simulink model "rtwdemo_advisor3"  (Simulink 7.6)
settings: Solver=FixedStepDiscrete  SolverMode=SingleTasking  StartTime=0.0  StopTime=4  FixedStep=1  RelTol=1e-3  AbsTol=1e-6
libraries: rtwdemowidgets x1
Description:
  | Using Model Advisor for optimizing the model for real-time deployment
settings Model: Creator=The MathWorks Inc.  CovMetricSettings=d  ExtModeTrigMode=oneshot  ExtModeArmWhenConnect=off  ExtModeAutoUpdateStatusClock=off
settings MATStruct: SampleTime=1  Offset=0  Priority=[20.0]
settings DataIOCC: LimitDataPoints=off  SaveOutput=off  SaveTime=off  SignalLoggingName=sigsOut
settings OptimizationCC: InlineParams=on  InlineInvariantSignals=on  PassReuseOutputArgsAs=Individual arguments  ZeroExternalMemoryAtStartup=off  ZeroInternalMemoryAtStartup=off  NoFixptDivByZeroProtection=on  EfficientFloat2IntCast=on  EfficientMapNaN2IntZero=off  OptimizeModelRefInitCode=on  LifeSpan=1
settings DebuggingCC: CheckExecutionContextPreStartOutputMsg=on  CheckExecutionContextRuntimeOutputMsg=on  SolverPrmCheckMsg=none  IntegerOverflowMsg=none  ParameterDowncastMsg=warning  ParameterOverflowMsg=warning  ParameterPrecisionLossMsg=none  StrictBusMsg=ErrorOnBusTreatedAsVector
settings HardwareCC: ProdIntDivRoundTo=Zero  ProdEndianess=LittleEndian  ProdHWDeviceType=Generic->32-bit Embedded Processor  TargetHWDeviceType=Generic->32-bit Embedded Processor
settings RTWCC: SystemTargetFile=ert.tlc  GenCodeOnly=on  TemplateMakefile=ert_default_tmf  GenerateReport=on  RTWVerbose=off  ProcessScript=ert_make_rtw_hook  IncludeHyperlinkInReport=on  LaunchReport=on
settings CodeAppCC: IgnoreCustomStorageClasses=off  IgnoreTestpoints=on  IncHierarchyInIds=on  IncDataTypeInIds=on
settings ERTTargetCC: TargetFcnLib=ansi_tfl_tmw.mat  MultiwordLength=2048  GenerateSampleERTMain=on  SupportNonFinite=off  ERTCustomFileTemplate=example_file_process.tlc  ConvertIfToSwitch=off

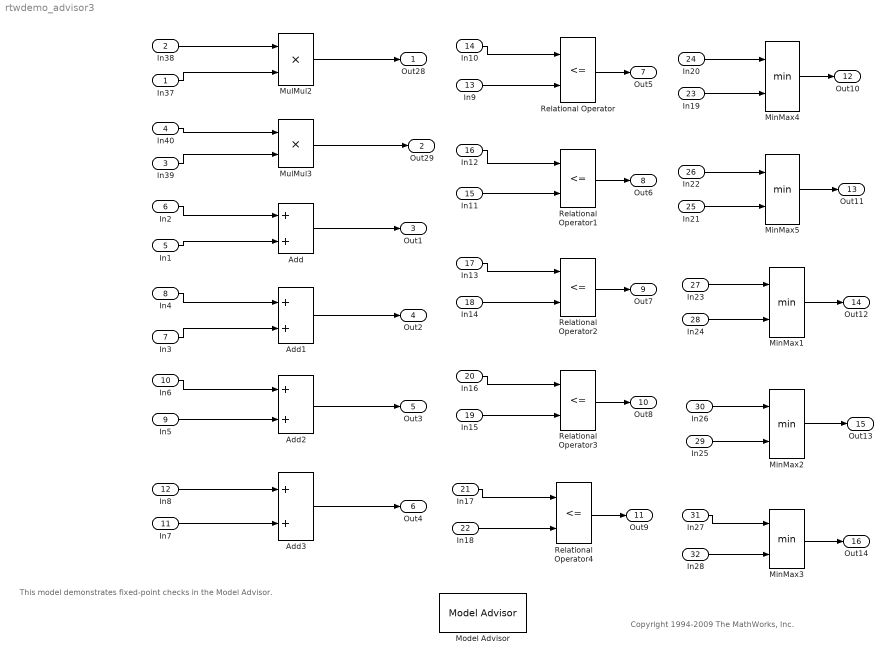
== system rtwdemo_advisor3 ==
  note: This model demonstrates fixed-point
      | checks in the Model Advisor.
  note: Copyright 1994-2009 The MathWorks, Inc.
  In37 : Inport  OutDataTypeStr=fixdt(1, 16, 1.375*2^-10, 0)  PortDimensions=1  SampleTime=1  Interpolate=off
  In38 : Inport  Port=2  OutDataTypeStr=fixdt(1, 16, 1.25 * 2^-10, 0)  PortDimensions=1  SampleTime=1  Interpolate=off
  In39 : Inport  Port=3  OutDataTypeStr=fixdt(1,16,10)  PortDimensions=1  SampleTime=1  Interpolate=off
  In40 : Inport  Port=4  OutDataTypeStr=fixdt(1, 16, 2^-10,1)  PortDimensions=1  SampleTime=1  Interpolate=off
  In1 : Inport  Port=5  OutDataTypeStr=fixdt(1,8,5)  PortDimensions=1  SampleTime=1  Interpolate=off
  In2 : Inport  Port=6  OutDataTypeStr=fixdt(1,16,8)  PortDimensions=1  SampleTime=1  Interpolate=off
  In3 : Inport  Port=7  OutDataTypeStr=fixdt(1,8,5)  PortDimensions=1  SampleTime=1  Interpolate=off
  In4 : Inport  Port=8  OutDataTypeStr=fixdt(0,8,8)  PortDimensions=1  SampleTime=1  Interpolate=off
  In5 : Inport  Port=9  OutDataTypeStr=fixdt(1, 8, 2^-5,6)  PortDimensions=1  SampleTime=1  Interpolate=off
  In6 : Inport  Port=10  OutDataTypeStr=fixdt(0,8,8)  PortDimensions=1  SampleTime=1  Interpolate=off
  In7 : Inport  Port=11  OutDataTypeStr=fixdt(1, 8, 1.5*2^-5, 0)  PortDimensions=1  SampleTime=1  Interpolate=off
  In8 : Inport  Port=12  OutDataTypeStr=fixdt(0,8,8)  PortDimensions=1  SampleTime=1  Interpolate=off
  In9 : Inport  Port=13  OutDataTypeStr=fixdt(1,8,5)  PortDimensions=1  SampleTime=1  Interpolate=off
  In10 : Inport  Port=14  OutDataTypeStr=fixdt(1,16,8)  PortDimensions=1  SampleTime=1  Interpolate=off
  In11 : Inport  Port=15  OutDataTypeStr=fixdt(1,8,5)  PortDimensions=1  SampleTime=1  Interpolate=off
  In12 : Inport  Port=16  OutDataTypeStr=fixdt(0,16,8)  PortDimensions=1  SampleTime=1  Interpolate=off
  In13 : Inport  Port=17  OutDataTypeStr=fixdt(1,8,5)  PortDimensions=1  SampleTime=1  Interpolate=off
  In14 : Inport  Port=18  OutDataTypeStr=fixdt(0,16,8)  PortDimensions=1  SampleTime=1  Interpolate=off
  In15 : Inport  Port=19  OutDataTypeStr=fixdt(1, 8, 1.125*2^-5, 0)  PortDimensions=1  SampleTime=1  Interpolate=off
  In16 : Inport  Port=20  OutDataTypeStr=fixdt(1,16,8)  PortDimensions=1  SampleTime=1  Interpolate=off
  In17 : Inport  Port=21  OutDataTypeStr=fixdt(1, 8, 1.125*2^-5, 0)  PortDimensions=1  SampleTime=1  Interpolate=off
  In18 : Inport  Port=22  OutDataTypeStr=fixdt(1,16,8)  PortDimensions=1  SampleTime=1  Interpolate=off
  In19 : Inport  Port=23  OutDataTypeStr=fixdt(1,8,5)  PortDimensions=1  SampleTime=1  Interpolate=off
  In20 : Inport  Port=24  OutDataTypeStr=fixdt(1,16,8)  PortDimensions=1  SampleTime=1  Interpolate=off
  In21 : Inport  Port=25  OutDataTypeStr=fixdt(1,8,5)  PortDimensions=1  SampleTime=1  Interpolate=off
  In22 : Inport  Port=26  OutDataTypeStr=fixdt(0,16,8)  PortDimensions=1  SampleTime=1  Interpolate=off
  In23 : Inport  Port=27  OutDataTypeStr=fixdt(1,8,5)  PortDimensions=1  SampleTime=1  Interpolate=off
  In24 : Inport  Port=28  OutDataTypeStr=fixdt(0,16,8)  PortDimensions=1  SampleTime=1  Interpolate=off
  In25 : Inport  Port=29  OutDataTypeStr=fixdt(1, 8, 1.125*2^-5, 0)  PortDimensions=1  SampleTime=1  Interpolate=off
  In26 : Inport  Port=30  OutDataTypeStr=fixdt(1,16,8)  PortDimensions=1  SampleTime=1  Interpolate=off
  In27 : Inport  Port=31  OutDataTypeStr=fixdt(1, 8, 1.125*2^-5, 0)  PortDimensions=1  SampleTime=1  Interpolate=off
  In28 : Inport  Port=32  OutDataTypeStr=fixdt(1,16,8)  PortDimensions=1  SampleTime=1  Interpolate=off
  Add : Sum  OutDataTypeStr=fixdt(1,16,10)
  Add1 : Sum  OutDataTypeStr=fixdt(0,16,10)
  Add2 : Sum  OutDataTypeStr=fixdt(0,16,10)
  Add3 : Sum  OutDataTypeStr=fixdt(0,16,10)
  MinMax{1..5} (5 alike) : MinMax  Inputs=2  ZeroCross=off
  Model Advisor : rtwdemowidgets/Model Advisor  SystemSampleTime=-1  attrib_overrides={}
  MulMul2 : Product  OutDataTypeStr=fixdt(1, 16, 1.5*2^-10, 0)
  MulMul3 : Product  OutDataTypeStr=fixdt(1,16,10)
  Relational Operator{,1..4} (5 alike) : RelationalOperator  Operator=<=  OutDataTypeStr=uint(8)  ZeroCross=off
  Out28 : Outport
  Out29 : Outport  Port=2
  Out1 : Outport  Port=3
  Out2 : Outport  Port=4
  Out3 : Outport  Port=5
  Out4 : Outport  Port=6
  Out5 : Outport  Port=7
  Out6 : Outport  Port=8
  Out7 : Outport  Port=9
  Out8 : Outport  Port=10
  Out9 : Outport  Port=11
  Out10 : Outport  Port=12
  Out11 : Outport  Port=13
  Out12 : Outport  Port=14
  Out13 : Outport  Port=15
  Out14 : Outport  Port=16
  wires:
  In37/1 -> MulMul2/2
  MulMul2/1 -> Out28/1
  In38/1 -> MulMul2/1
  In39/1 -> MulMul3/2
  MulMul3/1 -> Out29/1
  In40/1 -> MulMul3/1
  In1/1 -> Add/2
  Add/1 -> Out1/1
  In2/1 -> Add/1
  In3/1 -> Add1/2
  Add1/1 -> Out2/1
  In4/1 -> Add1/1
  In5/1 -> Add2/2
  Add2/1 -> Out3/1
  In6/1 -> Add2/1
  In7/1 -> Add3/2
  Add3/1 -> Out4/1
  In8/1 -> Add3/1
  In9/1 -> Relational Operator/2
  Relational Operator/1 -> Out5/1
  In10/1 -> Relational Operator/1
  In11/1 -> Relational Operator1/2
  Relational Operator1/1 -> Out6/1
  In12/1 -> Relational Operator1/1
  Relational Operator2/1 -> Out7/1
  In14/1 -> Relational Operator2/2
  In13/1 -> Relational Operator2/1
  In15/1 -> Relational Operator3/2
  Relational Operator3/1 -> Out8/1
  In16/1 -> Relational Operator3/1
  Relational Operator4/1 -> Out9/1
  In17/1 -> Relational Operator4/1
  In18/1 -> Relational Operator4/2
  In19/1 -> MinMax4/2
  MinMax4/1 -> Out10/1
  In20/1 -> MinMax4/1
  In21/1 -> MinMax5/2
  MinMax5/1 -> Out11/1
  In22/1 -> MinMax5/1
  MinMax1/1 -> Out12/1
  In24/1 -> MinMax1/2
  In23/1 -> MinMax1/1
  In25/1 -> MinMax2/2
  MinMax2/1 -> Out13/1
  In26/1 -> MinMax2/1
  MinMax3/1 -> Out14/1
  In27/1 -> MinMax3/1
  In28/1 -> MinMax3/2
